simulink model "gm_soc_dvbs2_fpga"  (R2025b)
settings: Solver=VariableStepAuto  StartTime=0.0  StopTime=10.0  RelTol=1e-3
InitFcn:
  | soc_dvbs2_init;
undefined symbols (not defined in the file or in its folder): Add, coefficientsLog, coefficientsSqrt1, coefficientsSqrt2, dataBits, Deinterleaver, designMultirateFIR, noisePow, Shift, Short, soc_dvbs2_designFIRFilter, soc_dvbs2_txPacketBits, syncWord, txDataOut, txFiltCoeff, XData
libraries: simulink x304, hdlsllib x265, dspsigops x15, dsphdlfiltering2 x8, hdlmdlgenlib x6, dsphdlsigops2 x5, commseqgen3 x5, dsphdlmathfun2 x3, hwlogicconnlib x2, whdledac x2, commhdlcrc x2, whdlutilities x1
(part 29 of 36)

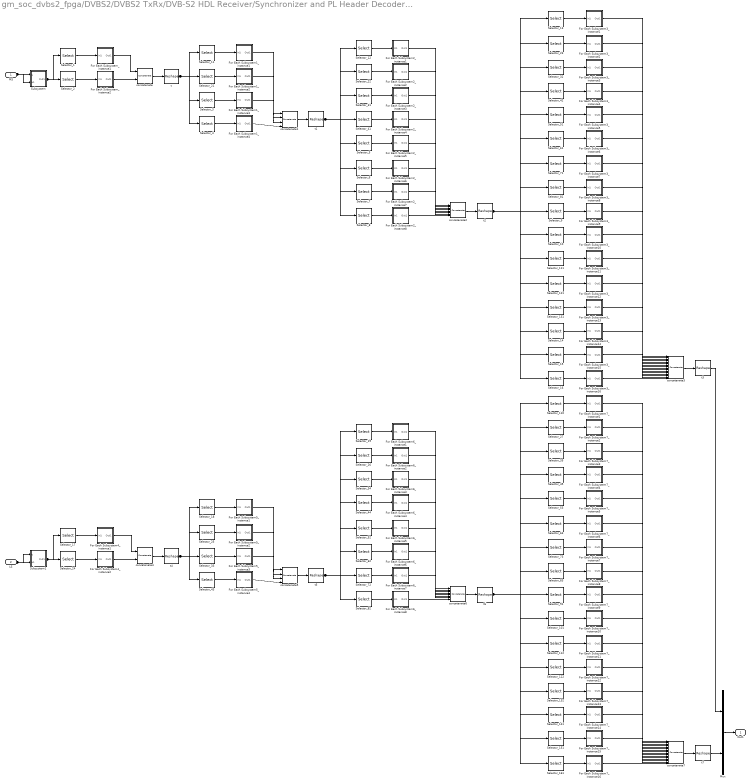
== system gm_soc_dvbs2_fpga/DVBS2/DVBS2 TxRx/DVB-S2 HDL Receiver/Synchronizer and PL Header Decoder/PL Header Recovery/PL Header Decoder/ML Decoder/Integer to Bit Convertor ==
  MS : Inport  OutDataTypeStr=uint32  PortDimensions=1  SampleTime=2.5e-07
  LS : Inport  Port=2  OutDataTypeStr=uint32  PortDimensions=1  SampleTime=2.5e-07
  For Each Subsystem1_instance1 : Subsystem
  For Each Subsystem1_instance2 : Subsystem
  For Each Subsystem1_instance3 : Subsystem
  For Each Subsystem1_instance4 : Subsystem
  For Each Subsystem2_instance1 : Subsystem
  For Each Subsystem2_instance2 : Subsystem
  For Each Subsystem2_instance3 : Subsystem
  For Each Subsystem2_instance4 : Subsystem
  For Each Subsystem2_instance5 : Subsystem
  For Each Subsystem2_instance6 : Subsystem
  For Each Subsystem2_instance7 : Subsystem
  For Each Subsystem2_instance8 : Subsystem
  For Each Subsystem3_instance1 : Subsystem
  For Each Subsystem3_instance10 : Subsystem
  For Each Subsystem3_instance11 : Subsystem
  For Each Subsystem3_instance12 : Subsystem
  For Each Subsystem3_instance13 : Subsystem
  For Each Subsystem3_instance14 : Subsystem
  For Each Subsystem3_instance15 : Subsystem
  For Each Subsystem3_instance16 : Subsystem
  For Each Subsystem3_instance2 : Subsystem
  For Each Subsystem3_instance3 : Subsystem
  For Each Subsystem3_instance4 : Subsystem
  For Each Subsystem3_instance5 : Subsystem
  For Each Subsystem3_instance6 : Subsystem
  For Each Subsystem3_instance7 : Subsystem
  For Each Subsystem3_instance8 : Subsystem
  For Each Subsystem3_instance9 : Subsystem
  For Each Subsystem4_instance1 : Subsystem
  For Each Subsystem4_instance2 : Subsystem
  For Each Subsystem5_instance1 : Subsystem
  For Each Subsystem5_instance2 : Subsystem
  For Each Subsystem5_instance3 : Subsystem
  For Each Subsystem5_instance4 : Subsystem
  For Each Subsystem6_instance1 : Subsystem
  For Each Subsystem6_instance2 : Subsystem
  For Each Subsystem6_instance3 : Subsystem
  For Each Subsystem6_instance4 : Subsystem
  For Each Subsystem6_instance5 : Subsystem
  For Each Subsystem6_instance6 : Subsystem
  For Each Subsystem6_instance7 : Subsystem
  For Each Subsystem6_instance8 : Subsystem
  For Each Subsystem7_instance1 : Subsystem
  For Each Subsystem7_instance10 : Subsystem
  For Each Subsystem7_instance11 : Subsystem
  For Each Subsystem7_instance12 : Subsystem
  For Each Subsystem7_instance13 : Subsystem
  For Each Subsystem7_instance14 : Subsystem
  For Each Subsystem7_instance15 : Subsystem
  For Each Subsystem7_instance16 : Subsystem
  For Each Subsystem7_instance2 : Subsystem
  For Each Subsystem7_instance3 : Subsystem
  For Each Subsystem7_instance4 : Subsystem
  For Each Subsystem7_instance5 : Subsystem
  For Each Subsystem7_instance6 : Subsystem
  For Each Subsystem7_instance7 : Subsystem
  For Each Subsystem7_instance8 : Subsystem
  For Each Subsystem7_instance9 : Subsystem
  For Each Subsystem_instance1 : Subsystem
  For Each Subsystem_instance2 : Subsystem
  Mux : Mux  Inputs=2
  Selector_1 : Selector  InputPortWidth=2  IndexOptions=Index vector (dialog)  Indices=double(1)  OutputSizes=1
  Selector_10 : Selector  InputPortWidth=16  IndexOptions=Index vector (dialog)  Indices=double(10)  OutputSizes=1
  Selector_101 : Selector  InputPortWidth=16  IndexOptions=Index vector (dialog)  Indices=double(10)  OutputSizes=1
  Selector_11 : Selector  InputPortWidth=4  IndexOptions=Index vector (dialog)  Indices=double(1)  OutputSizes=1
  Selector_110 : Selector  InputPortWidth=16  IndexOptions=Index vector (dialog)  Indices=double(1)  OutputSizes=1
  Selector_111 : Selector  InputPortWidth=16  IndexOptions=Index vector (dialog)  Indices=double(11)  OutputSizes=1
  Selector_112 : Selector  InputPortWidth=16  IndexOptions=Index vector (dialog)  Indices=double(11)  OutputSizes=1
  Selector_12 : Selector  InputPortWidth=8  IndexOptions=Index vector (dialog)  Indices=double(1)  OutputSizes=1
  Selector_121 : Selector  InputPortWidth=16  IndexOptions=Index vector (dialog)  Indices=double(12)  OutputSizes=1
  Selector_122 : Selector  InputPortWidth=16  IndexOptions=Index vector (dialog)  Indices=double(12)  OutputSizes=1
  Selector_13 : Selector  InputPortWidth=16  IndexOptions=Index vector (dialog)  Indices=double(1)  OutputSizes=1
  Selector_131 : Selector  InputPortWidth=16  IndexOptions=Index vector (dialog)  Indices=double(13)  OutputSizes=1
  Selector_132 : Selector  InputPortWidth=16  IndexOptions=Index vector (dialog)  Indices=double(13)  OutputSizes=1
  Selector_14 : Selector  InputPortWidth=16  IndexOptions=Index vector (dialog)  Indices=double(14)  OutputSizes=1
  Selector_141 : Selector  InputPortWidth=16  IndexOptions=Index vector (dialog)  Indices=double(14)  OutputSizes=1
  Selector_15 : Selector  InputPortWidth=16  IndexOptions=Index vector (dialog)  Indices=double(15)  OutputSizes=1
  Selector_151 : Selector  InputPortWidth=16  IndexOptions=Index vector (dialog)  Indices=double(15)  OutputSizes=1
  Selector_16 : Selector  InputPortWidth=16  IndexOptions=Index vector (dialog)  Indices=double(16)  OutputSizes=1
  Selector_161 : Selector  InputPortWidth=16  IndexOptions=Index vector (dialog)  Indices=double(16)  OutputSizes=1
  Selector_17 : Selector  InputPortWidth=2  IndexOptions=Index vector (dialog)  Indices=double(1)  OutputSizes=1
  Selector_18 : Selector  InputPortWidth=4  IndexOptions=Index vector (dialog)  Indices=double(1)  OutputSizes=1
  Selector_19 : Selector  InputPortWidth=8  IndexOptions=Index vector (dialog)  Indices=double(1)  OutputSizes=1
  Selector_2 : Selector  InputPortWidth=2  IndexOptions=Index vector (dialog)  Indices=double(2)  OutputSizes=1
  Selector_21 : Selector  InputPortWidth=4  IndexOptions=Index vector (dialog)  Indices=double(2)  OutputSizes=1
  Selector_22 : Selector  InputPortWidth=8  IndexOptions=Index vector (dialog)  Indices=double(2)  OutputSizes=1
  Selector_23 : Selector  InputPortWidth=16  IndexOptions=Index vector (dialog)  Indices=double(2)  OutputSizes=1
  Selector_24 : Selector  InputPortWidth=2  IndexOptions=Index vector (dialog)  Indices=double(2)  OutputSizes=1
  Selector_25 : Selector  InputPortWidth=4  IndexOptions=Index vector (dialog)  Indices=double(2)  OutputSizes=1
  Selector_26 : Selector  InputPortWidth=8  IndexOptions=Index vector (dialog)  Indices=double(2)  OutputSizes=1
  Selector_27 : Selector  InputPortWidth=16  IndexOptions=Index vector (dialog)  Indices=double(2)  OutputSizes=1
  Selector_3 : Selector  InputPortWidth=4  IndexOptions=Index vector (dialog)  Indices=double(3)  OutputSizes=1
  Selector_31 : Selector  InputPortWidth=8  IndexOptions=Index vector (dialog)  Indices=double(3)  OutputSizes=1
  Selector_32 : Selector  InputPortWidth=16  IndexOptions=Index vector (dialog)  Indices=double(3)  OutputSizes=1
  Selector_33 : Selector  InputPortWidth=4  IndexOptions=Index vector (dialog)  Indices=double(3)  OutputSizes=1
  Selector_34 : Selector  InputPortWidth=8  IndexOptions=Index vector (dialog)  Indices=double(3)  OutputSizes=1
  Selector_35 : Selector  InputPortWidth=16  IndexOptions=Index vector (dialog)  Indices=double(3)  OutputSizes=1
  Selector_4 : Selector  InputPortWidth=4  IndexOptions=Index vector (dialog)  Indices=double(4)  OutputSizes=1
  Selector_41 : Selector  InputPortWidth=8  IndexOptions=Index vector (dialog)  Indices=double(4)  OutputSizes=1
  Selector_42 : Selector  InputPortWidth=16  IndexOptions=Index vector (dialog)  Indices=double(4)  OutputSizes=1
  Selector_43 : Selector  InputPortWidth=4  IndexOptions=Index vector (dialog)  Indices=double(4)  OutputSizes=1
  Selector_44 : Selector  InputPortWidth=8  IndexOptions=Index vector (dialog)  Indices=double(4)  OutputSizes=1
  Selector_45 : Selector  InputPortWidth=16  IndexOptions=Index vector (dialog)  Indices=double(4)  OutputSizes=1
  Selector_5 : Selector  InputPortWidth=8  IndexOptions=Index vector (dialog)  Indices=double(5)  OutputSizes=1
  Selector_51 : Selector  InputPortWidth=16  IndexOptions=Index vector (dialog)  Indices=double(5)  OutputSizes=1
  Selector_52 : Selector  InputPortWidth=8  IndexOptions=Index vector (dialog)  Indices=double(5)  OutputSizes=1
  Selector_53 : Selector  InputPortWidth=16  IndexOptions=Index vector (dialog)  Indices=double(5)  OutputSizes=1
  Selector_6 : Selector  InputPortWidth=8  IndexOptions=Index vector (dialog)  Indices=double(6)  OutputSizes=1
  Selector_61 : Selector  InputPortWidth=16  IndexOptions=Index vector (dialog)  Indices=double(6)  OutputSizes=1
  Selector_62 : Selector  InputPortWidth=8  IndexOptions=Index vector (dialog)  Indices=double(6)  OutputSizes=1
  Selector_63 : Selector  InputPortWidth=16  IndexOptions=Index vector (dialog)  Indices=double(6)  OutputSizes=1
  Selector_7 : Selector  InputPortWidth=8  IndexOptions=Index vector (dialog)  Indices=double(7)  OutputSizes=1
  Selector_71 : Selector  InputPortWidth=16  IndexOptions=Index vector (dialog)  Indices=double(7)  OutputSizes=1
  Selector_72 : Selector  InputPortWidth=8  IndexOptions=Index vector (dialog)  Indices=double(7)  OutputSizes=1
  Selector_73 : Selector  InputPortWidth=16  IndexOptions=Index vector (dialog)  Indices=double(7)  OutputSizes=1
  Selector_8 : Selector  InputPortWidth=8  IndexOptions=Index vector (dialog)  Indices=double(8)  OutputSizes=1
  Selector_81 : Selector  InputPortWidth=16  IndexOptions=Index vector (dialog)  Indices=double(8)  OutputSizes=1
  Selector_82 : Selector  InputPortWidth=8  IndexOptions=Index vector (dialog)  Indices=double(8)  OutputSizes=1
  Selector_83 : Selector  InputPortWidth=16  IndexOptions=Index vector (dialog)  Indices=double(8)  OutputSizes=1
  Selector_9 : Selector  InputPortWidth=16  IndexOptions=Index vector (dialog)  Indices=double(9)  OutputSizes=1
  Selector_91 : Selector  InputPortWidth=16  IndexOptions=Index vector (dialog)  Indices=double(9)  OutputSizes=1
  Subsystem : Subsystem
  Subsystem1 : Subsystem
  concatenate : Concatenate
  concatenate1 : Concatenate  NumInputs=4
  concatenate2 : Concatenate  NumInputs=8
  concatenate3 : Concatenate  NumInputs=16
  concatenate4 : Concatenate
  concatenate5 : Concatenate  NumInputs=4
  concatenate6 : Concatenate  NumInputs=8
  concatenate7 : Concatenate  NumInputs=16
  t{,1..7} (8 alike) : Reshape
  Out1 : Outport  SampleTime=2.5e-07
  wires:
  Selector_73/1 -> For Each Subsystem7_instance7/1(In1)
  For Each Subsystem3_instance9/1(Out1) -> concatenate3/9
  Selector_110/1 -> For Each Subsystem7_instance1/1(In1)
  For Each Subsystem7_instance11/1(Out1) -> concatenate7/11
  Selector_45/1 -> For Each Subsystem7_instance4/1(In1)
  Selector_26/1 -> For Each Subsystem6_instance2/1(In1)
  Mux/1 -> Out1/1
  Selector_72/1 -> For Each Subsystem6_instance7/1(In1)
  Selector_19/1 -> For Each Subsystem6_instance1/1(In1)
  For Each Subsystem7_instance15/1(Out1) -> concatenate7/15
  For Each Subsystem6_instance3/1(Out1) -> concatenate6/3
  For Each Subsystem7_instance16/1(Out1) -> concatenate7/16
  For Each Subsystem2_instance2/1(Out1) -> concatenate2/2
  For Each Subsystem7_instance14/1(Out1) -> concatenate7/14
  Selector_27/1 -> For Each Subsystem7_instance2/1(In1)
  For Each Subsystem5_instance3/1(Out1) -> concatenate5/3
  Selector_24/1 -> For Each Subsystem4_instance2/1(In1)
  t5/1 -> Selector_72/1, Selector_62/1, Selector_52/1, Selector_34/1, Selector_26/1, Selector_19/1, Selector_44/1, Selector_82/1
  Selector_52/1 -> For Each Subsystem6_instance5/1(In1)
  For Each Subsystem7_instance8/1(Out1) -> concatenate7/8
  For Each Subsystem7_instance13/1(Out1) -> concatenate7/13
  Subsystem1/1(Out1) -> Selector_24/1, Selector_17/1
  For Each Subsystem7_instance10/1(Out1) -> concatenate7/10
  Selector_43/1 -> For Each Subsystem5_instance4/1(In1)
  t7/1 -> Mux/2
  For Each Subsystem7_instance12/1(Out1) -> concatenate7/12
  Selector_161/1 -> For Each Subsystem7_instance16/1(In1)
  For Each Subsystem7_instance9/1(Out1) -> concatenate7/9
  For Each Subsystem7_instance7/1(Out1) -> concatenate7/7
  For Each Subsystem7_instance6/1(Out1) -> concatenate7/6
  Selector_151/1 -> For Each Subsystem7_instance15/1(In1)
  For Each Subsystem7_instance5/1(Out1) -> concatenate7/5
  Selector_83/1 -> For Each Subsystem7_instance8/1(In1)
  concatenate4/1 -> t4/1
  For Each Subsystem7_instance4/1(Out1) -> concatenate7/4
  Selector_3/1 -> For Each Subsystem1_instance3/1(In1)
  concatenate5/1 -> t5/1
  For Each Subsystem7_instance3/1(Out1) -> concatenate7/3
  For Each Subsystem6_instance2/1(Out1) -> concatenate6/2
  For Each Subsystem7_instance2/1(Out1) -> concatenate7/2
  Selector_91/1 -> For Each Subsystem7_instance9/1(In1)
  Selector_6/1 -> For Each Subsystem2_instance6/1(In1)
  For Each Subsystem7_instance1/1(Out1) -> concatenate7/1
  For Each Subsystem3_instance6/1(Out1) -> concatenate3/6
  Selector_63/1 -> For Each Subsystem7_instance6/1(In1)
  t6/1 -> Selector_161/1, Selector_141/1, Selector_112/1, Selector_101/1, Selector_83/1, Selector_73/1, Selector_63/1, Selector_45/1, Selector_35/1, Selector_27/1, Selector_110/1, Selector_132/1, Selector_151/1, Selector_91/1, Selector_53/1, Selector_122/1
  Selector_132/1 -> For Each Subsystem7_instance13/1(In1)
  For Each Subsystem3_instance15/1(Out1) -> concatenate3/15
  Selector_25/1 -> For Each Subsystem5_instance2/1(In1)
  concatenate7/1 -> t7/1
  Selector_141/1 -> For Each Subsystem7_instance14/1(In1)
  Selector_18/1 -> For Each Subsystem5_instance1/1(In1)
  t4/1 -> Selector_43/1, Selector_33/1, Selector_18/1, Selector_25/1
  t3/1 -> Mux/1
  Selector_122/1 -> For Each Subsystem7_instance12/1(In1)
  Selector_62/1 -> For Each Subsystem6_instance6/1(In1)
  For Each Subsystem6_instance6/1(Out1) -> concatenate6/6
  For Each Subsystem6_instance8/1(Out1) -> concatenate6/8
  Selector_112/1 -> For Each Subsystem7_instance11/1(In1)
  Selector_101/1 -> For Each Subsystem7_instance10/1(In1)
  For Each Subsystem5_instance1/1(Out1) -> concatenate5/1
  Selector_44/1 -> For Each Subsystem6_instance4/1(In1)
  Selector_53/1 -> For Each Subsystem7_instance5/1(In1)
  Selector_35/1 -> For Each Subsystem7_instance3/1(In1)
  Selector_33/1 -> For Each Subsystem5_instance3/1(In1)
  For Each Subsystem3_instance1/1(Out1) -> concatenate3/1
  For Each Subsystem6_instance7/1(Out1) -> concatenate6/7
  For Each Subsystem6_instance5/1(Out1) -> concatenate6/5
  For Each Subsystem6_instance4/1(Out1) -> concatenate6/4
  For Each Subsystem6_instance1/1(Out1) -> concatenate6/1
  For Each Subsystem2_instance1/1(Out1) -> concatenate2/1
  concatenate6/1 -> t6/1
  Selector_82/1 -> For Each Subsystem6_instance8/1(In1)
  Selector_21/1 -> For Each Subsystem1_instance2/1(In1)
  For Each Subsystem4_instance2/1(Out1) -> concatenate4/2
  Selector_10/1 -> For Each Subsystem3_instance10/1(In1)
  LS/1 -> Subsystem1/2(u1), Subsystem1/1(u)
  Selector_34/1 -> For Each Subsystem6_instance3/1(In1)
  For Each Subsystem5_instance4/1(Out1) -> concatenate5/4
  For Each Subsystem5_instance2/1(Out1) -> concatenate5/2
  For Each Subsystem4_instance1/1(Out1) -> concatenate4/1
  Selector_17/1 -> For Each Subsystem4_instance1/1(In1)
  For Each Subsystem3_instance16/1(Out1) -> concatenate3/16
  For Each Subsystem3_instance14/1(Out1) -> concatenate3/14
  concatenate1/1 -> t1/1
  For Each Subsystem3_instance13/1(Out1) -> concatenate3/13
  For Each Subsystem3_instance12/1(Out1) -> concatenate3/12
  For Each Subsystem3_instance11/1(Out1) -> concatenate3/11
  Selector_41/1 -> For Each Subsystem2_instance4/1(In1)
  For Each Subsystem3_instance10/1(Out1) -> concatenate3/10
  For Each Subsystem3_instance8/1(Out1) -> concatenate3/8
  For Each Subsystem3_instance7/1(Out1) -> concatenate3/7
  For Each Subsystem3_instance5/1(Out1) -> concatenate3/5
  For Each Subsystem3_instance4/1(Out1) -> concatenate3/4
  For Each Subsystem3_instance3/1(Out1) -> concatenate3/3
  For Each Subsystem3_instance2/1(Out1) -> concatenate3/2
  concatenate3/1 -> t3/1
  Selector_16/1 -> For Each Subsystem3_instance16/1(In1)
  Selector_15/1 -> For Each Subsystem3_instance15/1(In1)
  For Each Subsystem2_instance5/1(Out1) -> concatenate2/5
  Selector_14/1 -> For Each Subsystem3_instance14/1(In1)
  Selector_131/1 -> For Each Subsystem3_instance13/1(In1)
  Selector_121/1 -> For Each Subsystem3_instance12/1(In1)
  Selector_111/1 -> For Each Subsystem3_instance11/1(In1)
  t/1 -> Selector_3/1, Selector_21/1, Selector_11/1, Selector_4/1
  Selector_9/1 -> For Each Subsystem3_instance9/1(In1)
  Selector_81/1 -> For Each Subsystem3_instance8/1(In1)
  Selector_71/1 -> For Each Subsystem3_instance7/1(In1)
  Selector_61/1 -> For Each Subsystem3_instance6/1(In1)
  Selector_51/1 -> For Each Subsystem3_instance5/1(In1)
  t1/1 -> Selector_7/1, Selector_5/1, Selector_41/1, Selector_31/1, Selector_22/1, Selector_6/1, Selector_12/1, Selector_8/1
  Selector_42/1 -> For Each Subsystem3_instance4/1(In1)
  Selector_32/1 -> For Each Subsystem3_instance3/1(In1)
  Selector_23/1 -> For Each Subsystem3_instance2/1(In1)
  Selector_13/1 -> For Each Subsystem3_instance1/1(In1)
  Selector_22/1 -> For Each Subsystem2_instance2/1(In1)
  For Each Subsystem2_instance8/1(Out1) -> concatenate2/8
  For Each Subsystem2_instance7/1(Out1) -> concatenate2/7
  For Each Subsystem2_instance6/1(Out1) -> concatenate2/6
  For Each Subsystem2_instance4/1(Out1) -> concatenate2/4
  For Each Subsystem2_instance3/1(Out1) -> concatenate2/3
  concatenate2/1 -> t2/1
  Selector_8/1 -> For Each Subsystem2_instance8/1(In1)
  Selector_7/1 -> For Each Subsystem2_instance7/1(In1)
  For Each Subsystem_instance2/1(Out1) -> concatenate/2
  Selector_5/1 -> For Each Subsystem2_instance5/1(In1)
  Selector_31/1 -> For Each Subsystem2_instance3/1(In1)
  Selector_12/1 -> For Each Subsystem2_instance1/1(In1)
  For Each Subsystem1_instance4/1(Out1) -> concatenate1/4
  For Each Subsystem1_instance3/1(Out1) -> concatenate1/3
  For Each Subsystem1_instance2/1(Out1) -> concatenate1/2
  MS/1 -> Subsystem/2(u1), Subsystem/1(u)
  For Each Subsystem1_instance1/1(Out1) -> concatenate1/1
  Selector_4/1 -> For Each Subsystem1_instance4/1(In1)
  Selector_11/1 -> For Each Subsystem1_instance1/1(In1)
  For Each Subsystem_instance1/1(Out1) -> concatenate/1
  concatenate/1 -> t/1
  Selector_2/1 -> For Each Subsystem_instance2/1(In1)
  Selector_1/1 -> For Each Subsystem_instance1/1(In1)
  t2/1 -> Selector_16/1, Selector_15/1, Selector_14/1, Selector_131/1, Selector_121/1, Selector_111/1, Selector_10/1, Selector_9/1, Selector_81/1, Selector_71/1, Selector_61/1, Selector_51/1, Selector_42/1, Selector_32/1, Selector_13/1, Selector_23/1
  Subsystem/1(Out1) -> Selector_2/1, Selector_1/1

== system gm_soc_dvbs2_fpga/DVBS2/DVBS2 TxRx/DVB-S2 HDL Receiver/Synchronizer and PL Header Decoder/Time Frequency and Coarse Phase Synchronizer/Coarse Phase Synchronizer/Coarse Phase Corrector/Reciprocal ==
  dataIn : Inport  OutDataTypeStr=fixdt(1, 13, 10)  PortDimensions=1  SampleTime=2.5e-07
  Compare To Constant : simulink/Logic and Bit Operations/Compare To Constant  relop=<  const=0  OutDataTypeStr=boolean
  Data Type Conversion : DataTypeConversion  OutDataTypeStr=fixdt(1,WL,0)  ConvertRealWorld=Stored Integer (SI)  SaturateOnIntegerOverflow=off  RndMeth=Floor
  Data Type Conversion1 : DataTypeConversion  OutDataTypeStr=fixdt(0,LUTAddrWL,0)  ConvertRealWorld=Stored Integer (SI)  SaturateOnIntegerOverflow=off  RndMeth=Floor
  Data Type Conversion2 : DataTypeConversion  OutDataTypeStr=fixdt(0,WL-LUTAddrWL,0)  ConvertRealWorld=Stored Integer (SI)  SaturateOnIntegerOverflow=off  RndMeth=Floor
  Delay : Delay  DelayLength=1
  Delay1 : Delay  DelayLength=1
  Delay2 : Delay  DelayLength=1
  Extract Bits : simulink/Logic and Bit Operations/Extract Bits  bitsToExtract=Range ending with least significant bit  numBits=LUTAddrWL  bitIdxRange=[0 7]  outScalingMode=Treat bit field as an integer
  Function Impl : Subsystem
  dataOut : Outport  SampleTime=2.5e-07
  wires:
  Delay1/1 -> Data Type Conversion2/1
  dataIn/1 -> Data Type Conversion/1
  Data Type Conversion2/1 -> Function Impl/1(switch)
  Compare To Constant/1 -> Delay1/1
  Data Type Conversion/1 -> Delay/1
  Delay2/1 -> Data Type Conversion1/1
  Delay/1 -> Extract Bits/1, Compare To Constant/1
  Extract Bits/1 -> Delay2/1
  Data Type Conversion1/1 -> Function Impl/2(LUTAddr)
  Function Impl/1(functionValues) -> dataOut/1

== system gm_soc_dvbs2_fpga/DVBS2/DVBS2 TxRx/DVB-S2 HDL Receiver/Synchronizer and PL Header Decoder/Time Frequency and Coarse Phase Synchronizer/Fine Frequency Synchronizer/Modified L and R Algorithm/L and R Algorithm 18 point ==
  z : Inport  OutDataTypeStr=fixdt(1, 18, 13)  PortDimensions=1  SampleTime=2.5e-07
      settings: SignalType=complex
  zvalid : Inport  Port=2  OutDataTypeStr=boolean  PortDimensions=1  SampleTime=2.5e-07
  Add : Sum  Inputs=+++  OutDataTypeStr=fixdt(1, 38, 22)
  Compute R(m) for 1 to 6 : Subsystem  mask{m=reshape(double([1;2;3;4;5;6]), [1  6])}
      mask prompts: m "m values for computing R(m):"
  Compute R(m) for 13 to 18 : Subsystem  mask{m=reshape(double([13;14;15;16;17;18]), [1  6])}
      mask prompts: m "m values for computing R(m):"
  Compute R(m) for 7 to 12 : Subsystem  mask{m=reshape(double([7;8;9;10;11;12]), [1  6])}
      mask prompts: m "m values for computing R(m):"
  Data Type Conversion : DataTypeConversion  OutDataTypeStr=fixdt(1,16,11)  SaturateOnIntegerOverflow=off  RndMeth=Floor
  Delay{1..6} (6 alike) : Delay
  dataIn : Outport  SampleTime=2.5e-07
  wires:
  Delay4/1 -> Add/2
  z/1 -> Data Type Conversion/1
  Compute R(m) for 13 to 18/1(sum) -> Delay5/1
  Compute R(m) for 7 to 12/1(sum) -> Delay4/1
  Data Type Conversion/1 -> Delay3/1
  zvalid/1 -> Delay1/1
  Delay1/1 -> Compute R(m) for 1 to 6/2(zvalid), Compute R(m) for 13 to 18/2(zvalid), Compute R(m) for 7 to 12/2(zvalid)
  Delay3/1 -> Compute R(m) for 1 to 6/1(z), Compute R(m) for 13 to 18/1(z), Compute R(m) for 7 to 12/1(z)
  Compute R(m) for 1 to 6/1(sum) -> Delay2/1
  Delay2/1 -> Add/1
  Add/1 -> Delay6/1
  Delay5/1 -> Add/3
  Delay6/1 -> dataIn/1

== system gm_soc_dvbs2_fpga/DVBS2/DVBS2 TxRx/DVB-S2 HDL Receiver/Synchronizer and PL Header Decoder/Time Frequency and Coarse Phase Synchronizer/Fine Frequency Synchronizer/Modified L and R Algorithm/Moving Average ==
  dataIn : Inport  OutDataTypeStr=fixdt(1, 38, 22)  PortDimensions=1  SampleTime=2.5e-07
      settings: SignalType=complex
  validIn : Inport  Port=2  OutDataTypeStr=boolean  PortDimensions=1  SampleTime=2.5e-07
  Add : Sum  OutDataTypeStr=fixdt(1, 53, 36)  AccumDataTypeStr=fixdt(1, 54, 36)  SampleTime=2.5e-07
  Add1 : Sum  Inputs=+-  OutDataTypeStr=fixdt(1, 39, 22)  AccumDataTypeStr=fixdt(1, 39, 22)  SampleTime=2.5e-07
  Data Type Conversion1 : DataTypeConversion  OutDataTypeStr=fixdt(1, 53, 36)  SampleTime=2.5e-07  SaturateOnIntegerOverflow=off  RndMeth=Floor
  Delay : Delay  DelayLength=double(512)  InitialCondition="fi(0,1,38,22,\"hex\",\"0000000000\")"  ShowEnablePort=on
      settings: InputPortMap=u0,e6
  Delay1 : Delay  DelayLength=double(1)  InitialCondition="fi(0,1,53,36,\"hex\",\"00000000000000\")"  ShowEnablePort=on
      settings: InputPortMap=u0,e6
  Delay2 : Delay  DelayLength=double(2)  InitialCondition=0  SampleTime=2.5e-07
  Delay3 : Delay  DelayLength=double(2)  InitialCondition=0  SampleTime=2.5e-07
  Delay{4..8} (5 alike) : Delay  DelayLength=double(1)  InitialCondition=0  SampleTime=2.5e-07
  Gain : Gain  Gain="fi(0,0,9,9,\"hex\",\"001\")"  ParamDataTypeStr=fixdt(0, 9, 9)  OutDataTypeStr=fixdt(1, 53, 36)  SampleTime=2.5e-07
  dataOut : Outport  SampleTime=2.5e-07
  validOut : Outport  Port=2  SampleTime=2.5e-07
  wires:
  dataIn/1 -> Delay5/1, Delay/1
  Delay5/1 -> Add1/1
  Add1/1 -> Data Type Conversion1/1
  Delay7/1 -> Delay2/1
  Delay/1 -> Delay6/1
  validIn/1 -> Delay7/1, Delay/2
  Delay2/1 -> Delay1/2, Delay8/1
  Delay6/1 -> Add1/2
  Delay8/1 -> validOut/1
  Data Type Conversion1/1 -> Delay3/1
  Delay3/1 -> Gain/1
  Gain/1 -> Add/1
  Delay1/1 -> Add/2
  Add/1 -> Delay1/1, Delay4/1
  Delay4/1 -> dataOut/1

== system gm_soc_dvbs2_fpga/DVBS2/DVBS2 TxRx/DVB-S2 HDL Receiver/Synchronizer and PL Header Decoder/Time Frequency and Coarse Phase Synchronizer/Fine Gain Control/Reciprocal/Function Impl ==
  switch : Inport  OutDataTypeStr=fixdt(0, 1, 0)  PortDimensions=1  SampleTime=2.5e-07
  LUTAddr : Inport  Port=2  OutDataTypeStr=fixdt(0, 12, 0)  PortDimensions=1  SampleTime=2.5e-07
  Delay{6..8,10,15..16} (6 alike) : Delay
  Delay9 : Delay  DelayLength=1
  LUT1 : LookupNDDirect  NumberOfTableDimensions=1  Table=LUT(:,1)  DiagnosticForOutOfRangeInput=Error
  LUT2 : LookupNDDirect  NumberOfTableDimensions=1  Table=LUT(:,2)  DiagnosticForOutOfRangeInput=Error
  Multiport Switch : MultiPortSwitch  DataPortOrder=Zero-based contiguous  Inputs=2  zeroidx=on  OutDataTypeStr=fixdt(1, 26, 14)  SaturateOnIntegerOverflow=off  InputSameDT=off
  functionValues : Outport  SampleTime=2.5e-07
  wires:
  LUT1/1 -> Delay16/1
  Delay8/1 -> Delay10/1
  LUTAddr/1 -> Delay7/1, Delay6/1
  Delay6/1 -> LUT1/1
  LUT2/1 -> Delay15/1
  Delay10/1 -> Multiport Switch/1
  Delay7/1 -> LUT2/1
  Delay16/1 -> Multiport Switch/3
  switch/1 -> Delay8/1
  Delay15/1 -> Multiport Switch/2
  Multiport Switch/1 -> Delay9/1
  Delay9/1 -> functionValues/1

== system gm_soc_dvbs2_fpga/DVBS2/DVBS2 TxRx/DVB-S2 HDL Receiver/Synchronizer and PL Header Decoder/Time Frequency and Coarse Phase Synchronizer/Time and Coarse Frequency Synchronizer/Coarse Frequency Estimator/Direct Digital Synthesis ==
  v : Inport  OutDataTypeStr=fixdt(1, 37, 26)  PortDimensions=1  SampleTime=2.5e-07
  rst : Inport  Port=2  OutDataTypeStr=boolean  PortDimensions=1  SampleTime=2.5e-07
  Constant : Constant  Value=true  OutDataTypeStr=boolean  SampleTime=-1
  Data Type Conversion : DataTypeConversion  OutDataTypeStr=fixdt(1,21,21)  SaturateOnIntegerOverflow=off  RndMeth=Floor
  Data Type Conversion1 : DataTypeConversion  OutDataTypeStr=fixdt(1,21,0)  ConvertRealWorld=Stored Integer (SI)  SaturateOnIntegerOverflow=off  RndMeth=Floor
  Delay1 : Delay
  Delay14 : Delay
  Delay2 : Delay  DelayLength=1  InitialCondition=0
  Gain : Gain  Gain=1/config.SamplesPerSymbol  ParamDataTypeStr=fixdt(0,2,2)  OutDataTypeStr=fixdt(1, 37, 26)
  NCO HDL Optimized : dsphdlsigops2/NCO  PhaseIncrementSource=Input port  PhaseIncrement=100  PhaseOffsetSource=Property  PhaseOffset=0  DitherSource=None  NumDitherBits=11  SamplesPerFrame=1  LUTCompress=off  ResetAction=on  Waveform=Complex exponential  PhasePort=off  SimulateUsing=Code generation  AccumulatorWL=21  PhaseQuantization=on  NumQuantizerAccumulatorBits=14  OutputDataType=Binary point scaling  OutputWL=16  OutputFL=14
  NCO HDL Optimized_term1 : Terminator
  Repeat : dspsigops/Repeat  FactorSource=Dialog parameter  N=config.SamplesPerSymbol  Nmax=16  RateOptions=Allow multirate processing  ic=0  mode=Unused parameter value
  Repeat1 : dspsigops/Repeat  FactorSource=Dialog parameter  N=config.SamplesPerSymbol  Nmax=16  RateOptions=Allow multirate processing  ic=0  mode=Unused parameter value
  complexEst : Outport  SampleTime=6.25e-08
  normalizedEst : Outport  Port=2  SampleTime=2.5e-07
  wires:
  v/1 -> Delay14/1
  NCO HDL Optimized/2 -> NCO HDL Optimized_term1/1
  rst/1 -> Repeat1/1
  Data Type Conversion1/1 -> Repeat/1
  Gain/1 -> Delay1/1
  Delay14/1 -> Gain/1
  Repeat/1 -> NCO HDL Optimized/1
  Data Type Conversion/1 -> Data Type Conversion1/1, normalizedEst/1
  Delay1/1 -> Data Type Conversion/1
  Repeat1/1 -> NCO HDL Optimized/2
  Constant/1 -> NCO HDL Optimized/3
  NCO HDL Optimized/1 -> Delay2/1
  Delay2/1 -> complexEst/1

== system gm_soc_dvbs2_fpga/DVBS2/DVBS2 TxRx/DVB-S2 HDL Receiver/Synchronizer and PL Header Decoder/Time Frequency and Coarse Phase Synchronizer/Time and Coarse Frequency Synchronizer/Coarse Frequency Estimator/Frequency Error Detector ==
  dataIn : Inport  OutDataTypeStr=fixdt(1, 18, 13)  PortDimensions=1  SampleTime=2.5e-07
      settings: SignalType=complex
  pilotIdx : Inport  Port=2  OutDataTypeStr=fixdt(0, 11, 0)  PortDimensions=1  SampleTime=2.5e-07
  pilotValid : Inport  Port=3  OutDataTypeStr=boolean  PortDimensions=1  SampleTime=2.5e-07
  Compare To Constant1 : simulink/Logic and Bit Operations/Compare To Constant  relop=<=  const=config.PilotMaxIdx - 2  OutDataTypeStr=boolean
  Compare To Constant2 : simulink/Logic and Bit Operations/Compare To Constant  relop=>=  const=config.PilotMinIdx + 2  OutDataTypeStr=boolean
  Complex Multiplier : Subsystem
  Complex to Real-Imag : ComplexToRealImag  Output=Imag
  Delay{,1..11,16..19,24} (17 alike) : Delay
  Delay12 : Delay  DelayLength=1
  Delay13 : Delay  DelayLength=1
  Delay14 : Delay  DelayLength=1
  Delay15 : Delay  DelayLength=8
  Gain : Gain  Gain=conj(config.Pilot)  OutDataTypeStr=fixdt(1, 18, 13)
      mask init:
      | Simulink.suppressDiagnostic(gcb, 'SimulinkFixedPoint:util:fxpParameterPrecisionLoss');
  Gain1 : Gain  Gain=config.Pilot  OutDataTypeStr=fixdt(1, 18, 13)
      mask init:
      | Simulink.suppressDiagnostic(gcb, 'SimulinkFixedPoint:util:fxpParameterPrecisionLoss');
  Logical Operator : Logic  Inputs=3  AllPortsSameDT=off  OutDataTypeStr=boolean
  Math Function : Math  Operator=conj  OutDataTypeStr=fixdt(1, 18, 13)
  Unit Delay Enabled Synchronous : hdlsllib/Discrete/Unit Delay Enabled Synchronous  InitialCondition=0.0  SampleTime=-1
  e : Outport  SampleTime=2.5e-07
  wires:
  Delay6/1 -> Delay7/1
  Delay5/1 -> Delay19/1
  dataIn/1 -> Delay24/1, Delay/1
  Delay1/1 -> Gain1/1
  Delay24/1 -> Gain/1
  Delay/1 -> Math Function/1
  Gain/1 -> Delay4/1
  Compare To Constant2/1 -> Delay2/1
  Math Function/1 -> Delay1/1
  Delay15/1 -> Delay11/1
  pilotIdx/1 -> Compare To Constant2/1, Compare To Constant1/1
  Unit Delay Enabled Synchronous/1 -> Delay14/1
  Compare To Constant1/1 -> Delay18/1
  pilotValid/1 -> Delay3/1
  Delay4/1 -> Delay5/1
  Gain1/1 -> Delay6/1
  Delay2/1 -> Logical Operator/1
  Delay18/1 -> Logical Operator/2
  Delay3/1 -> Logical Operator/3
  Logical Operator/1 -> Delay8/1
  Delay19/1 -> Complex Multiplier/1(In1)
  Delay7/1 -> Delay17/1
  Delay8/1 -> Delay9/1
  Delay17/1 -> Complex Multiplier/2(In2)
  Delay9/1 -> Delay16/1
  Complex Multiplier/1(Out1) -> Delay10/1
  Delay16/1 -> Delay15/1
  Delay10/1 -> Complex to Real-Imag/1
  Complex to Real-Imag/1 -> Delay12/1
  Delay11/1 -> Delay13/1
  Delay12/1 -> Unit Delay Enabled Synchronous/1
  Delay13/1 -> Unit Delay Enabled Synchronous/2
  Delay14/1 -> e/1

== system gm_soc_dvbs2_fpga/DVBS2/DVBS2 TxRx/DVB-S2 HDL Receiver/Synchronizer and PL Header Decoder/Time Frequency and Coarse Phase Synchronizer/Time and Coarse Frequency Synchronizer/Coarse Frequency Estimator/Loop Filter ==
  e : Inport  OutDataTypeStr=fixdt(1, 37, 26)  PortDimensions=1  SampleTime=2.5e-07
  rst : Inport  Port=2  OutDataTypeStr=boolean  PortDimensions=1  SampleTime=2.5e-07
  En : Inport  Port=3  OutDataTypeStr=boolean  PortDimensions=1  SampleTime=2.5e-07
  Add : Sum  OutDataTypeStr=fixdt(1, 37, 26)  AccumDataTypeStr=fixdt(1, 38, 26)  SampleTime=2.5e-07
  Delay{,1..3} (4 alike) : Delay  DelayLength=double(1)  InitialCondition=0  SampleTime=2.5e-07
  Delay14 : Delay  DelayLength=double(2)  InitialCondition=0  SampleTime=2.5e-07
  Integrator Gain : Gain  Gain="fi(0,0,16,29,\"hex\",\"8582\")"  ParamDataTypeStr=fixdt(0, 16, 29)  OutDataTypeStr=fixdt(1, 37, 26)  SampleTime=2.5e-07
  Unit Delay Enabled Resettable Synchronous : hdlsllib/Discrete/Unit Delay Enabled Resettable Synchronous  InitialCondition=double(0)  SampleTime=-1
  v : Outport  SampleTime=2.5e-07
  rstOut : Outport  Port=2  SampleTime=2.5e-07
  wires:
  e/1 -> Delay14/1
  Delay/1 -> Delay3/1
  Delay14/1 -> Integrator Gain/1
  Delay1/1 -> Add/1
  Integrator Gain/1 -> Delay1/1
  En/1 -> Unit Delay Enabled Resettable Synchronous/2
  rst/1 -> Delay/1, Unit Delay Enabled Resettable Synchronous/3
  Unit Delay Enabled Resettable Synchronous/1 -> Delay2/1, Add/2
  Add/1 -> Unit Delay Enabled Resettable Synchronous/1
  Delay2/1 -> v/1
  Delay3/1 -> rstOut/1

== system gm_soc_dvbs2_fpga/DVBS2/DVBS2 TxRx/DVB-S2 HDL Receiver/Synchronizer and PL Header Decoder/Time Frequency and Coarse Phase Synchronizer/Time and Coarse Frequency Synchronizer/Coarse Frequency Estimator/Pilot Blks Counter ==
  pilotIdx : Inport  OutDataTypeStr=fixdt(0, 11, 0)  PortDimensions=1  SampleTime=2.5e-07
  pilotValid : Inport  Port=2  OutDataTypeStr=boolean  PortDimensions=1  SampleTime=2.5e-07
  rst : Inport  Port=3  OutDataTypeStr=boolean  PortDimensions=1  SampleTime=2.5e-07
  Compare To Constant : simulink/Logic and Bit Operations/Compare To Constant  relop===  const=config.PilotMinIdx  OutDataTypeStr=boolean
  HDL Counter : hdlsllib/Sources/HDL Counter  CountType=Free running  CountInit=0  CountStep=1  CountMax=25  CountFromType=Initial value  CountFrom=0  CountResetPort=on  CountLoadPort=off  CountEnbPort=on  CountDirPort=off  CountHitOutputPort=off  CountDataType=Unsigned  CountWordLen=16  CountFracLen=0  CountSampTime=1
  Logical Operator : Logic  AllPortsSameDT=off  OutDataTypeStr=boolean
  pilotBlkCount : Outport  SampleTime=2.5e-07
  wires:
  rst/1 -> HDL Counter/1
  pilotIdx/1 -> Compare To Constant/1
  Compare To Constant/1 -> Logical Operator/1
  HDL Counter/1 -> pilotBlkCount/1
  pilotValid/1 -> Logical Operator/2
  Logical Operator/1 -> HDL Counter/2

== system gm_soc_dvbs2_fpga/DVBS2/DVBS2 TxRx/DVB-S2 HDL Receiver/Synchronizer and PL Header Decoder/Time Frequency and Coarse Phase Synchronizer/Time and Coarse Frequency Synchronizer/Frame Synchronizer/Correlator ==
  note: Compute Energy
  note: Differential Detection
  dataIn : Inport  OutDataTypeStr=fixdt(1, 18, 13)  PortDimensions=1  SampleTime=2.5e-07
      settings: SignalType=complex
  validIn : Inport  Port=2  OutDataTypeStr=boolean  PortDimensions=1  SampleTime=2.5e-07
  Add4 : Sum  OutDataTypeStr=fixdt(1, 33, 30)
  Complex to Real-Imag : ComplexToRealImag  Output=Real
  Data Type Conversion : DataTypeConversion  OutDataTypeStr=fixdt(1,17,14)  SaturateOnIntegerOverflow=off  RndMeth=Floor
  Delay{,9..10,12} (4 alike) : Delay  DelayLength=1
  Delay{1..2,4..8,11,13..25} (21 alike) : Delay
  Delay3 : Delay  DelayLength=70-32
  Gain : Gain  Gain=fi(config.refSOFE,0,16,16)  OutDataTypeStr=fixdt(1,32,30)
  Gain1 : Gain  Gain=fi(config.refPLSCE,0,16,16)  OutDataTypeStr=fixdt(1,32,30)
  Math Function : Math  Operator=conj  OutDataTypeStr=fixdt(1, 18, 13)
  Math Function1 : Math  Operator=conj  OutDataTypeStr=fixdt(1, 18, 13)
  Moving Sum : Subsystem
  PLSC Correlator : Subsystem  mask{coefs=reshape(complex(double([0+0.017543859649122803i;0;0+0.017543859649122803i;0;0-0.017543859649122803i;0;0-0.017543859649122803i;0;0+0.017543859649122803i;0;0-0.017543859649122803i;0;0+0.017543859649122803i;0;0-0.017543859649122803i;0;0+0.017543859649122803i;0;0-0.017543859649122803i;0;0-0.017543859649122803i;0;0+0.017543859649122803i;0;0-0.017543859649122803i;0;0-0.017543859649122803i;0;0+0.017543859649122803i;0;0+0.017543859649122803i;0;0+0.017543859649122803i;0;0+0.017543859649122803i;0;0-0.017543859649122803i;0;0-0.017543859649122803i;0;0-0.017543859649122803i;0;0-0.017543859649122803i;0;0-0.017543859649122803i;0;0+0.017543859649122803i;0;0+0.017543859649122803i;0;0-0.017543859649122803i;0;0+0.017543859649122803i;0;0+0.017543859649122803i;0;0+0.017543859649122803i;0;0-0.017543859649122803i;0;0-0.017543859649122803i;0;0+0.017543859649122803i])), [1  63]), shareFactor=double(4)}
      mask prompts: coefs "Coefficients:"; shareFactor "Number of cycles:"
      mask init:
      | adjustDelay = double(62);
      | coefs = reshape(complex(double([0+0.017543859649122803i;0;0+0.017543859649122803i;0;0-0.017543859649122803i;0;0-0.017543859649122803i;0;0+0.017543859649122803i;0;0-0.017543859649122803i;0;0+0.017543859649122803i;0;0-0.017543859649122803i;0;0+0.017543859649122803i;0;0-0.017543859649122803i;0;0-0.017543859649122803i;0;0+0.017543859649122803i;0;0-0.017543859649122803i;0;0-0.017543859649122803i;0;0+0.017543859649122803i;0;0+0.017543859649122803i;0;0+0.017543859649122803i;0;0+0.017543859649122803i;0;0-0.017543859649122803i;0;0-0.017543859649122803i;0;0-0.017543859649122803i;0;0-0.017543859649122803i;0;0-0.017543859649122803i;0;0+0.017543859649122803i;0;0+0.017543859649122803i;0;0-0.017543859649122803i;0;0+0.017543859649122803i;0;0+0.017543859649122803i;0;0+0.017543859649122803i;0;0-0.017543859649122803i;0;0-0.017543859649122803i;0;0+0.017543859649122803i])), [1  63]);
      | directFormLatency = double(69);
      | partlySerialExtraDelay = double(1);
      | partlySerialLatency = double(27);
      | shareFactor = double(4);
  Product : Product  OutDataTypeStr=fixdt(1, 18, 13)
  Product1 : Product  OutDataTypeStr=fixdt(1, 18, 13)
  SOF Correlator : Subsystem  mask{coefs=reshape(complex(double([0-0.017543859649122803i;0+0.017543859649122803i;0+0.017543859649122803i;0-0.017543859649122803i;0+0.017543859649122803i;0-0.017543859649122803i;0-0.017543859649122803i;0+0.017543859649122803i;0-0.017543859649122803i;0-0.017543859649122803i;0+0.017543859649122803i;0+0.017543859649122803i;0-0.017543859649122803i;0+0.017543859649122803i;0+0.017543859649122803i;0+0.017543859649122803i;0-0.017543859649122803i;0+0.017543859649122803i;0+0.017543859649122803i;0+0.017543859649122803i;0+0.017543859649122803i;0-0.017543859649122803i;0-0.017543859649122803i;0-0.017543859649122803i;0-0.017543859649122803i])), [1  25]), shareFactor=double(4)}
      mask prompts: coefs "Coefficients:"; shareFactor "Number of cycles:"
      mask init:
      | adjustDelay = double(26);
      | coefs = reshape(complex(double([0-0.017543859649122803i;0+0.017543859649122803i;0+0.017543859649122803i;0-0.017543859649122803i;0+0.017543859649122803i;0-0.017543859649122803i;0-0.017543859649122803i;0+0.017543859649122803i;0-0.017543859649122803i;0-0.017543859649122803i;0+0.017543859649122803i;0+0.017543859649122803i;0-0.017543859649122803i;0+0.017543859649122803i;0+0.017543859649122803i;0+0.017543859649122803i;0-0.017543859649122803i;0+0.017543859649122803i;0+0.017543859649122803i;0+0.017543859649122803i;0+0.017543859649122803i;0-0.017543859649122803i;0-0.017543859649122803i;0-0.017543859649122803i;0-0.017543859649122803i])), [1  25]);
      | directFormLatency = double(31);
      | partlySerialExtraDelay = double(2);
      | partlySerialLatency = double(18);
      | shareFactor = double(4);
  SOFCorrOut : Outport  SampleTime=2.5e-07
  PLSCCorrOut : Outport  Port=2  SampleTime=2.5e-07
  threshold : Outport  Port=3  SampleTime=2.5e-07
  wires:
  Delay8/1 -> PLSC Correlator/2(validIn), SOF Correlator/2(validIn)
  dataIn/1 -> Delay1/1, Math Function1/1, Delay19/1
  Math Function/1 -> Delay24/1
  Delay1/1 -> Delay/1, Math Function/1
  Delay18/1 -> Product1/2
  Delay17/1 -> Delay21/1
  Delay/1 -> Delay23/1
  Moving Sum/2(E2) -> Add4/2
  Delay10/1 -> PLSCCorrOut/1
  Delay19/1 -> Product1/1
  Delay9/1 -> SOFCorrOut/1
  Math Function1/1 -> Delay18/1
  validIn/1 -> Delay2/1, Delay17/1
  Delay24/1 -> Delay4/1
  Delay23/1 -> Delay5/1
  Delay12/1 -> Data Type Conversion/1
  Moving Sum/1(E1) -> Add4/1
  Delay11/1 -> Delay25/1
  Delay2/1 -> Delay22/1
  Delay3/1 -> Delay9/1
  Product1/1 -> Delay20/1
  Delay4/1 -> Product/1
  Add4/1 -> Delay12/1
  PLSC Correlator/1(dataOut) -> Delay10/1
  Delay5/1 -> Product/2
  Delay22/1 -> Delay6/1
  Delay20/1 -> Complex to Real-Imag/1
  Delay21/1 -> Delay11/1
  Data Type Conversion/1 -> threshold/1
  Delay7/1 -> SOF Correlator/1(dataIn), PLSC Correlator/1(dataIn)
  Product/1 -> Delay7/1
  Complex to Real-Imag/1 -> Delay16/1, Delay15/1
  Delay6/1 -> Delay8/1
  Delay15/1 -> Gain/1
  Delay16/1 -> Gain1/1
  SOF Correlator/1(dataOut) -> Delay3/1
  Gain/1 -> Delay14/1
  Gain1/1 -> Delay13/1
  Delay25/1 -> Moving Sum/3(validIn)
  Delay14/1 -> Moving Sum/1(scaled1)
  Delay13/1 -> Moving Sum/2(scaled2)

== system gm_soc_dvbs2_fpga/DVBS2/DVBS2 TxRx/DVB-S2 HDL Receiver/Synchronizer and PL Header Decoder/Time Frequency and Coarse Phase Synchronizer/Time and Coarse Frequency Synchronizer/Frame Synchronizer/Pilot and Sync Pulse Indicator ==
  note: Compute Energy
  note: Compute Energy
  SOFCorrDelayed : Inport  OutDataTypeStr=fixdt(1, 15, 12)  PortDimensions=1  SampleTime=2.5e-07
      settings: SignalType=complex
  PLSCCorr : Inport  Port=2  OutDataTypeStr=fixdt(1, 15, 11)  PortDimensions=1  SampleTime=2.5e-07
      settings: SignalType=complex
  threshold : Inport  Port=3  OutDataTypeStr=fixdt(1, 15, 12)  PortDimensions=1  SampleTime=2.5e-07
  Bus Creator : BusCreator  Inputs=3
  Complex to Real-Imag : ComplexToRealImag  Output=Real
  Complex to Real-Imag1 : ComplexToRealImag  Output=Real
  Corr Add : Sum  OutDataTypeStr=fixdt(1, 17, 12)
  Corr Subtract : Sum  Inputs=+-  OutDataTypeStr=fixdt(1, 17, 12)
  Delay{1..10,15..16,19..21,24..26} (18 alike) : Delay  DelayLength=1
  Delay{11..14,17..18,22..23} (8 alike) : Delay
  Logical Operator : Logic  Operator=OR  AllPortsSameDT=off  OutDataTypeStr=boolean
  Math Function : Math  Operator=conj  OutDataTypeStr=fixdt(1, 17, 12)
  Math Function1 : Math  Operator=conj  OutDataTypeStr=fixdt(1, 17, 12)
  Product : Product  OutDataTypeStr=fixdt(1,18,15)
  Product1 : Product  OutDataTypeStr=fixdt(1,18,15)
  Relational Operator : RelationalOperator  Operator=>  OutDataTypeStr=boolean  RndMeth=Simplest  InputSameDT=off
  Relational Operator1 : RelationalOperator  Operator=>  OutDataTypeStr=boolean  RndMeth=Simplest  InputSameDT=off
  Threshold Scaling : Gain  Gain=config.Threshold  OutDataTypeStr=fixdt(1, 15, 12)
      mask init:
      | Simulink.suppressDiagnostic(gcb, 'SimulinkFixedPoint:util:fxpParameterPrecisionLoss');
  ThresholdLimiter : Subsystem
  hasPilots : Outport  SampleTime=2.5e-07
  thresholdExceeded : Outport  Port=2  SampleTime=2.5e-07
  VisualizeCorrelationSignals : Outport  Port=3
  wires:
  threshold/1 -> Delay21/1
  Delay1/1 -> Delay8/1
  SOFCorrDelayed/1 -> Delay4/1, Delay2/1
  PLSCCorr/1 -> Delay5/1, Delay3/1
  Product/1 -> Delay11/1
  Delay5/1 -> Corr Subtract/2
  Delay3/1 -> Corr Add/2
  Delay2/1 -> Corr Add/1
  Delay4/1 -> Corr Subtract/1
  Relational Operator1/1 -> Logical Operator/2
  Corr Add/1 -> Delay15/1, Delay16/1
  Corr Subtract/1 -> Delay20/1, Delay19/1
  Delay16/1 -> Delay13/1
  Delay15/1 -> Math Function/1
  Delay21/1 -> Delay24/1
  Delay20/1 -> Delay17/1
  Delay19/1 -> Math Function1/1
  Delay13/1 -> Product/1
  Math Function/1 -> Delay14/1
  Delay24/1 -> Delay22/1
  Bus Creator/1 -> VisualizeCorrelationSignals/1
  Math Function1/1 -> Delay18/1
  Delay14/1 -> Product/2
  Delay22/1 -> Threshold Scaling/1
  Delay17/1 -> Product1/1
  Delay9/1 -> hasPilots/1
  Delay18/1 -> Product1/2
  Delay26/1 -> Bus Creator/3, Relational Operator1/2, Relational Operator/2  "Threshold"
  Threshold Scaling/1 -> Delay23/1
  Delay25/1 -> ThresholdLimiter/1(x)
  Product1/1 -> Delay12/1
  Delay11/1 -> Complex to Real-Imag/1
  Delay23/1 -> Delay25/1
  Delay12/1 -> Complex to Real-Imag1/1
  Complex to Real-Imag/1 -> Delay6/1
  Relational Operator/1 -> Logical Operator/1, Delay9/1
  Complex to Real-Imag1/1 -> Delay1/1
  Delay6/1 -> Delay7/1
  ThresholdLimiter/1(y) -> Delay26/1
  Delay7/1 -> Bus Creator/1, Relational Operator/1  "PeakValueWithPilots"
  Delay8/1 -> Bus Creator/2, Relational Operator1/1  "PeakValueWithoutPilots"
  Logical Operator/1 -> Delay10/1
  Delay10/1 -> thresholdExceeded/1

== system gm_soc_dvbs2_fpga/DVBS2/DVBS2 TxRx/DVB-S2 HDL Receiver/Synchronizer and PL Header Decoder/Time Frequency and Coarse Phase Synchronizer/Time and Coarse Frequency Synchronizer/PL Data Descrambler and Pilot Valid Indicator/PL Data Descrambler ==
  reset : Inport  OutDataTypeStr=boolean  PortDimensions=1  SampleTime=2.5e-07
  inputCount : Inport  Port=2  OutDataTypeStr=uint32  PortDimensions=1  SampleTime=2.5e-07
  validIn : Inport  Port=3  OutDataTypeStr=boolean  PortDimensions=1  SampleTime=2.5e-07
  dataIn : Inport  Port=4  OutDataTypeStr=fixdt(1, 18, 13)  PortDimensions=1  SampleTime=2.5e-07
      settings: SignalType=complex
  Compare To Constant : simulink/Logic and Bit Operations/Compare To Constant  relop=<=  const="fi(0,0,32,0,\"hex\",\"0000003f\")"  OutDataTypeStr=boolean
  Delay1 : Delay  DelayLength=double(7)  InitialCondition=0  SampleTime=2.5e-07
  Delay{2..6,8,10..12,22..23} (11 alike) : Delay  DelayLength=double(1)  InitialCondition=0  SampleTime=2.5e-07
  Delay{13..21} (9 alike) : Delay  DelayLength=double(2)  InitialCondition=0  SampleTime=2.5e-07
  Delay7_absorbed : Delay  DelayLength=0
  Delay9 : Delay  DelayLength=double(7)  InitialCondition=0  SampleTime=2.5e-07
  Math Function : Math  Operator=conj  OutDataTypeStr=fixdt(1, 2, 0)
  PL Scramble Sequence Mapper LUT : Subsystem
  PL Scrambler Gold Sequence Generator : Subsystem  mask{n=double(0)}
      mask prompts: n "Index of Gold Sequence :"
  Product : Product  Inputs=**  OutDataTypeStr=fixdt(1, 18, 13)  SampleTime=2.5e-07
  Switch : Switch  Criteria=u2 ~= 0  Threshold="fi(0,0,1,0,\"hex\",\"0\")"  OutDataTypeStr=fixdt(1, 18, 13)  SampleTime=2.5e-07  SaturateOnIntegerOverflow=off  InputSameDT=off
  dataOut : Outport  SampleTime=2.5e-07
  validOut : Outport  Port=2  SampleTime=2.5e-07
  wires:
  PL Scrambler Gold Sequence Generator/1(dataOut) -> Delay2/1
  validIn/1 -> PL Scrambler Gold Sequence Generator/2(validIn)
  reset/1 -> PL Scrambler Gold Sequence Generator/1(reset)
  dataIn/1 -> Delay9/1
  Switch/1 -> Delay22/1
  inputCount/1 -> Delay1/1
  PL Scrambler Gold Sequence Generator/2(validOut) -> Delay5/1
  Delay5/1 -> Delay8/1
  Delay2/1 -> PL Scramble Sequence Mapper LUT/1(In1)
  Delay8/1 -> Delay17/1
  Delay1/1 -> Delay3/1
  Delay9/1 -> Delay6/1, Delay4/1
  Delay22/1 -> dataOut/1
  PL Scramble Sequence Mapper LUT/1(Out1) -> Delay7_absorbed/1
  Delay17/1 -> Delay21/1
  Delay3/1 -> Delay11/1
  Product/1 -> Delay20/1
  Delay4/1 -> Delay10/1
  Delay7_absorbed/1 -> Math Function/1
  Delay21/1 -> Delay23/1
  Delay6/1 -> Delay12/1
  Delay11/1 -> Compare To Constant/1
  Delay10/1 -> Delay15/1
  Math Function/1 -> Delay16/1
  Delay23/1 -> validOut/1
  Delay12/1 -> Delay13/1
  Compare To Constant/1 -> Delay14/1
  Delay15/1 -> Product/1
  Delay16/1 -> Product/2
  Delay13/1 -> Delay18/1
  Delay14/1 -> Delay19/1
  Delay18/1 -> Switch/1
  Delay19/1 -> Switch/2
  Delay20/1 -> Switch/3
